simulink model "RK_sim"  (R2020a)
settings: Solver=VariableStepAuto  StartTime=0.0  StopTime=2000  MaxStep=0.05  RelTol=1e-3
undefined symbols (not defined in the file or in its folder): magnitude
settings Model: Creator=stepanletyagin  LastModifiedBy=stepanletyagin
settings DataIOCC: ReturnWorkspaceOutputs=off

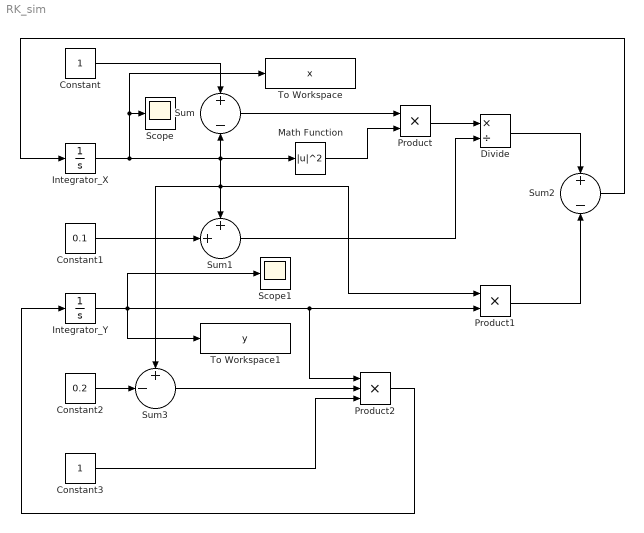
== system RK_sim ==
  Constant : Constant
  Constant1 : Constant  Value=0.1
  Constant2 : Constant  Value=0.2
  Constant3 : Constant
  Divide : Product  Inputs=*/
  Integrator_X : Integrator  InitialCondition=0.3
  Integrator_Y : Integrator  InitialCondition=0.3
  Math Function : Math  Operator=magnitude^2  SaturateOnIntegerOverflow=on
  Product : Product
  Product1 : Product
  Product2 : Product  Inputs=3
  Scope : Scope
  Scope1 : Scope
  Sum : Sum  Inputs=+-
  Sum1 : Sum  Inputs=++|
  Sum2 : Sum  Inputs=+-
  Sum3 : Sum  Inputs=+-|
  To Workspace : ToWorkspace  VariableName=x  SaveFormat=Timeseries  SampleTime=-1
      settings: Save2DSignal=2-D array (concatenate along first dimension)
  To Workspace1 : ToWorkspace  VariableName=y  SaveFormat=Timeseries  SampleTime=-1
      settings: Save2DSignal=2-D array (concatenate along first dimension)
  wires:
  Constant/1 -> Sum/1
  Sum/1 -> Product/1
  Math Function/1 -> Product/2
  Product/1 -> Divide/1
  Integrator_X/1 -> Scope/1, To Workspace/1, Product1/1, Sum3/1, Sum1/1, Math Function/1, Sum/2
  Constant1/1 -> Sum1/2
  Sum1/1 -> Divide/2
  Integrator_Y/1 -> Scope1/1, To Workspace1/1, Product2/1, Product1/2
  Product1/1 -> Sum2/2
  Divide/1 -> Sum2/1
  Sum2/1 -> Integrator_X/1
  Constant2/1 -> Sum3/2
  Sum3/1 -> Product2/2
  Constant3/1 -> Product2/3
  Product2/1 -> Integrator_Y/1
